simulink model "LIPMobsv"  (R2018b)
settings: Solver=VariableStepAuto  StartTime=0.0  StopTime=10.0  RelTol=1e-3
values from neighbouring files (symbols this model uses):
  arm_radius = leg_radius    (= 0.01)    [Nao_paramter.m]
  foot_height = 0.02    [Nao_paramter.m]
  foot_length = 0.1    [Nao_paramter.m]
  foot_mass = 0.17184    [Nao_paramter.m]
  foot_width = 0.05    [Nao_paramter.m]
  ground_height = 0.0025    [Nao_paramter.m]
  ground_length = 5    [Nao_paramter.m]
  ground_width = 2    [Nao_paramter.m]
  hand_mass = 0.18533    [Nao_paramter.m]
  head_mass = 0.60533    [Nao_paramter.m]
  hip_mass = 0.14053    [Nao_paramter.m]
  hip_off_Y = 0.05    [Nao_paramter.m]
  hip_off_Z = 0.085    [Nao_paramter.m]
  leg_radius = 0.01    [Nao_paramter.m]
  lowerarm_length = 0.05595    [Nao_paramter.m]
  lowerarm_mass = 0.07761    [Nao_paramter.m]
  neck_length = 0.03    [Nao_paramter.m]
  neck_mass = 0.07842    [Nao_paramter.m]
  neck_off_Z = 0.1265    [Nao_paramter.m]
  shoulder_mass = 0.09304    [Nao_paramter.m]
  thigh_mass = 0.38968    [Nao_paramter.m]
  tibia_mass = 0.30142    [Nao_paramter.m]
  torso_height = foot_height + tibia_length + thigh_length + 0.5*hip_off_Z    (= 0.2654)    [Nao_paramter.m]
  torso_mass = 1.0496    [Nao_paramter.m]
  upperarm_length = 0.105    [Nao_paramter.m]
  upperarm_mass = 0.15777    [Nao_paramter.m]
undefined symbols (not defined in the file or in its folder): sigbuilder_block, X, Y, Z
libraries: sm_lib x166, nesl_utility x34, Contact_Forces_Lib x20
(part 1 of 6)
settings Model: Creator=zicho  LastModifiedBy=zicho

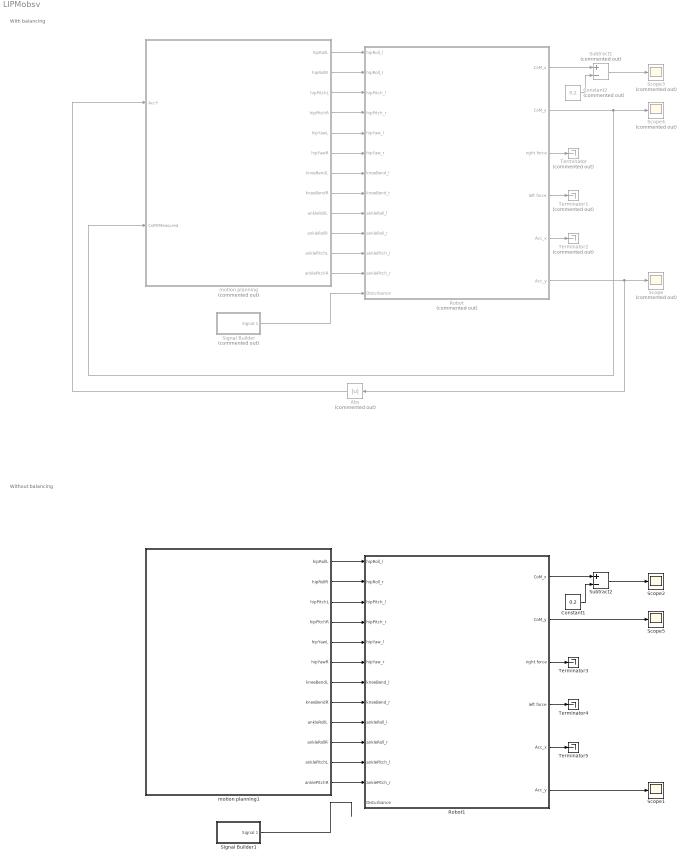
== system LIPMobsv ==
  note: With balancing
  note: Without balancing
  Abs : Abs  Commented=on
  Constant1 : Constant  Value=0.2
  Constant2 : Constant  Commented=on  Value=0.2
  Robot : Subsystem  Commented=on
      mask Display: image('multibody.jpg');
  Robot1 : Subsystem
      mask Display: image('multibody.jpg');
  Scope : Scope  Commented=on
  Scope1 : Scope
  Scope2 : Scope
  Scope3 : Scope  Commented=on
  Scope4 : Scope  Commented=on
  Scope5 : Scope
  Signal Builder : Subsystem  Tag=STV Subsys  Commented=on  LoadFcn=sigbuilder_block('load');  StartFcn=sigbuilder_block('start');  StopFcn=sigbuilder_block('stop');  ClipboardFcn=sigbuilder_block('clipboard');  mask(Sigbuilder block){tuvar=[0:10]}
      mask help: Simulink:masks:SigbuilderBlock_MD
      mask init:
      | if ~strcmp(get_param(bdroot(gcbh),'SimulationStatus'),'stopped') tuvar = sigbuilder_block('maskInit'); end
      settings: CopyFcn=sigbuilder_block('copy');  DeleteFcn=sigbuilder_block('delete');  ModelCloseFcn=sigbuilder_block('modelClose');  PreSaveFcn=sigbuilder_block('preSave');  PauseFcn=sigbuilder_block('pause');  ContinueFcn=sigbuilder_block('continue');  NameChangeFcn=sigbuilder_block('namechange');  OpenFcn=sigbuilder_block('open',[437.6 199.2 550.4 400 ]);  CloseFcn=sigbuilder_block('close');
      mask Display: plot(0, 0, 100, 100,[2, 2, 32, 32, 2], [68, 8, 8, 68, 68],[32, 2], [38, 38], [32, 19, 2],[53, 60, 44], [32, 17, 17, 2],[16, 16, 31, 31]);txt = getActiveGroup(gcbh);text(2, 100, txt,'verticalAlignment', 'top');
  Signal Builder1 : Subsystem  Tag=STV Subsys  LoadFcn=sigbuilder_block('load');  StartFcn=sigbuilder_block('start');  StopFcn=sigbuilder_block('stop');  ClipboardFcn=sigbuilder_block('clipboard');  mask(Sigbuilder block){tuvar=[0:10]}
      mask help: Simulink:masks:SigbuilderBlock_MD
      mask init:
      | if ~strcmp(get_param(bdroot(gcbh),'SimulationStatus'),'stopped') tuvar = sigbuilder_block('maskInit'); end
      settings: CopyFcn=sigbuilder_block('copy');  DeleteFcn=sigbuilder_block('delete');  ModelCloseFcn=sigbuilder_block('modelClose');  PreSaveFcn=sigbuilder_block('preSave');  PauseFcn=sigbuilder_block('pause');  ContinueFcn=sigbuilder_block('continue');  NameChangeFcn=sigbuilder_block('namechange');  OpenFcn=sigbuilder_block('open',[437.6 199.2 550.4 400 ]);  CloseFcn=sigbuilder_block('close');
      mask Display: plot(0, 0, 100, 100,[2, 2, 32, 32, 2], [68, 8, 8, 68, 68],[32, 2], [38, 38], [32, 19, 2],[53, 60, 44], [32, 17, 17, 2],[16, 16, 31, 31]);txt = getActiveGroup(gcbh);text(2, 100, txt,'verticalAlignment', 'top');
  Subtract1 : Sum  Commented=on  Inputs=+-
  Subtract2 : Sum  Inputs=+-
  Terminator : Terminator  Commented=on
  Terminator1 : Terminator  Commented=on
  Terminator2 : Terminator  Commented=on
  Terminator3 : Terminator
  Terminator4 : Terminator
  Terminator5 : Terminator
  motion planning : Stateflow chart  Commented=on  TreatAsAtomicUnit=on
  motion planning1 : Stateflow chart  TreatAsAtomicUnit=on
  wires:
  motion planning/8(kneeBendR) -> Robot/8(kneeBend_r)
  motion planning/5(hipYawL) -> Robot/5(hipYaw_l)
  motion planning/10(ankleRollR) -> Robot/10(ankleRoll_r)
  motion planning/11(anklePitchL) -> Robot/11(anklePitch_l)
  motion planning/9(ankleRollL) -> Robot/9(ankleRoll_l)
  motion planning/1(hipRollL) -> Robot/1(hipRoll_l)
  motion planning/2(hipRollR) -> Robot/2(hipRoll_r)
  motion planning/12(anklePitchR) -> Robot/12(anklePitch_r)
  motion planning/4(hipPitchR) -> Robot/4(hipPitch_r)
  motion planning/7(kneeBendL) -> Robot/7(kneeBend_l)
  motion planning/6(hipYawR) -> Robot/6(hipYaw_r)
  motion planning/3(hipPitchL) -> Robot/3(hipPitch_l)
  Robot/2(CoM_y) -> motion planning/2(CoMYMeasured), Scope4/1
  Robot/1(CoM_x) -> Subtract1/1
  Constant2/1 -> Subtract1/2
  Subtract1/1 -> Scope3/1
  Robot/3(right force) -> Terminator/1
  Robot/4(left force) -> Terminator1/1
  Signal Builder/1(Signal 1) -> Robot/13(Disturbance)
  Robot/6(Acc_y) -> Abs/1, Scope/1
  Robot/5(Acc_x) -> Terminator2/1
  Abs/1 -> motion planning/1(AccY)
  motion planning1/1(hipRollL) -> Robot1/1(hipRoll_l)
  motion planning1/2(hipRollR) -> Robot1/2(hipRoll_r)
  motion planning1/3(hipPitchL) -> Robot1/3(hipPitch_l)
  motion planning1/4(hipPitchR) -> Robot1/4(hipPitch_r)
  motion planning1/5(hipYawL) -> Robot1/5(hipYaw_l)
  motion planning1/6(hipYawR) -> Robot1/6(hipYaw_r)
  motion planning1/7(kneeBendL) -> Robot1/7(kneeBend_l)
  motion planning1/8(kneeBendR) -> Robot1/8(kneeBend_r)
  motion planning1/9(ankleRollL) -> Robot1/9(ankleRoll_l)
  motion planning1/10(ankleRollR) -> Robot1/10(ankleRoll_r)
  motion planning1/11(anklePitchL) -> Robot1/11(anklePitch_l)
  motion planning1/12(anklePitchR) -> Robot1/12(anklePitch_r)
  Subtract2/1 -> Scope2/1
  Constant1/1 -> Subtract2/2
  Robot1/6(Acc_y) -> Scope1/1
  Robot1/2(CoM_y) -> Scope5/1
  Robot1/1(CoM_x) -> Subtract2/1
  Robot1/3(right force) -> Terminator3/1
  Robot1/4(left force) -> Terminator4/1
  Robot1/5(Acc_x) -> Terminator5/1
  Signal Builder1/1(Signal 1) -> ?
